simulink model "car_system_SIL_PIL"  (R2019b)
settings: Solver=ode23tb  StartTime=0.0  StopTime=30  RelTol=1e-3
InitFcn:
  | CommonVariables
  | Klqr5Velocities
undefined symbols (not defined in the file): A_1, A_2, A_3, A_4, A_5, B1_1, B1_2, B1_3, B1_4, B1_5, BattChrgMax, BattDischrgMax, BrkPrsMax, ChrgLmt_bpt, Disabled, DischrgLmt_bpt, disk_abore, DLCXref, DLCYref, efficiency_table, F0z, h, Klqr1, Klqr2, Klqr3, Klqr4, Klqr5, MotSpd, MotTrq, mu_kinetic, Ndiff, num_pads, RegenBrkCutOff, RegenBrkSpd_bpt, Right, Rm, SOC_bpt, T_eff_bp, VEH, w_eff_bp
libraries: simulink x10, vehdynlibtire x8, vehdynlibsuspension x7, vehdynlibscenariocommon x5, autolibutils x4, sim3dlib x4, autolibmappedmotor x4, autolibshared x2, sharedtransform x2, vehdynlibviscommon x2, vehdynlibdriver x1, vehdynlibsteering x1
(part 4 of 7)

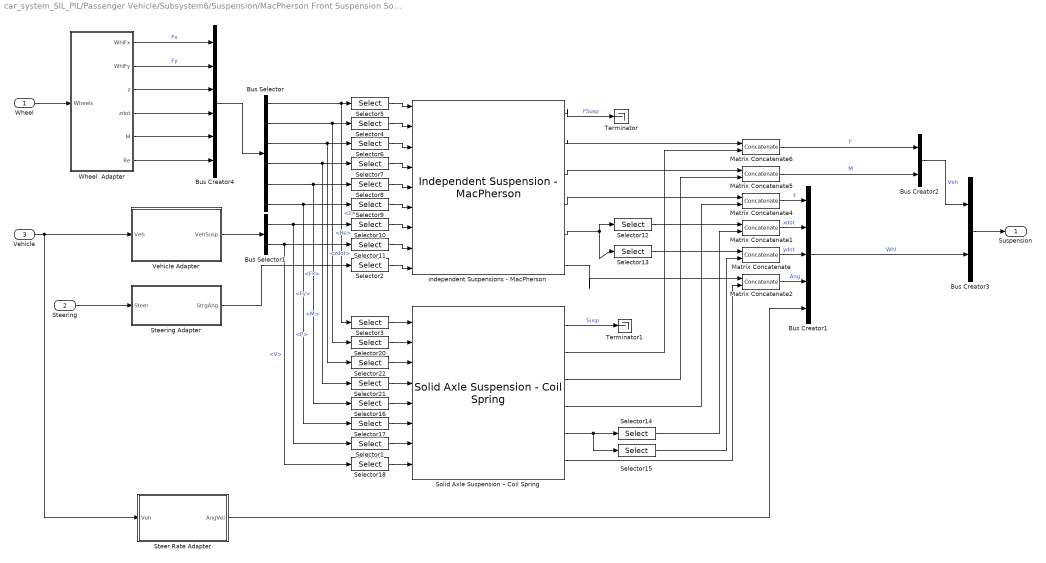
== system car_system_SIL_PIL/Passenger Vehicle/Subsystem6/Suspension/MacPherson Front Suspension Solid Axle Rear Suspension ==
  Wheel : Inport
  Steering : Inport  Port=2
  Vehicle : Inport  Port=3
  Bus Creator1 : BusCreator  Inputs=5
  Bus Creator2 : BusCreator  Inputs=2
  Bus Creator3 : BusCreator  Inputs=2
  Bus Creator4 : BusCreator  Inputs=6
  Bus Selector : BusSelector  OutputSignals=z,Re,zdot,Fx,Fy,M
  Bus Selector1 : BusSelector  OutputSignals=P,V
  Matrix Concatenate{,1..2,4..6} (6 alike) : Concatenate  Mode=Multidimensional array  ConcatenateDimension=2
  Selector1 : Selector  NumberOfDimensions=2  IndexOptions=Select all,Index vector (dialog)  Indices=[1 2],[3 4]  OutputSizes=1,1
  Selector10 : Selector  NumberOfDimensions=2  IndexOptions=Select all,Index vector (dialog)  Indices=[1 2],[1 2]  OutputSizes=1,1
  Selector11 : Selector  NumberOfDimensions=2  IndexOptions=Select all,Index vector (dialog)  Indices=[1 2],[1 2]  OutputSizes=1,1
  Selector12 : Selector  NumberOfDimensions=2  InputPortWidth=3  IndexOptions=Index vector (dialog),Select all  Indices=1,1  OutputSizes=1,1
  Selector13 : Selector  NumberOfDimensions=2  InputPortWidth=3  IndexOptions=Index vector (dialog),Select all  Indices=2,1  OutputSizes=1,1
  Selector14 : Selector  NumberOfDimensions=2  InputPortWidth=3  IndexOptions=Index vector (dialog),Select all  Indices=1,1  OutputSizes=1,1
  Selector15 : Selector  NumberOfDimensions=2  InputPortWidth=3  IndexOptions=Index vector (dialog),Select all  Indices=2,1  OutputSizes=1,1
  Selector{3,16,20..22} (5 alike) : Selector  IndexOptions=Index vector (dialog)  Indices=[3 4]  OutputSizes=1
  Selector17 : Selector  NumberOfDimensions=2  IndexOptions=Select all,Index vector (dialog)  Indices=[1 2],[3 4]  OutputSizes=1,1
  Selector18 : Selector  NumberOfDimensions=2  IndexOptions=Select all,Index vector (dialog)  Indices=[1 2],[3 4]  OutputSizes=1,1
  Selector{2,4..8} (6 alike) : Selector  IndexOptions=Index vector (dialog)  Indices=[1 2]  OutputSizes=1
  Selector9 : Selector  NumberOfDimensions=2  IndexOptions=Select all,Index vector (dialog)  Indices=[1 2],[1 2]  OutputSizes=1,1
  Solid Axle Suspension – Coil Spring : vehdynlibsuspension/Solid Axle Suspension - Coil Spring  NumAxl=1  NumTracksByAxl=2  StrgEnByAxl=0  TrackNumVec="[1  2]"  AxleNumVec="[1  1]"  SuspTypesByAxle=[1]  SuspImage=suspsacoil.png  AxlIxx=AxlIxx  AxlM=AxlM  TrackCoords=[0 0;VEH.TrackWidth*[-1 1]/2;0 0]  SuspCoords=[0 0;VEH.TrackWidth*[-1 1]/2;0 0]  KzWhlAxl=KzWhlAxl  F0zWhlAxl=F0zWhlAxl  CzWhlAxl=CzWhlAxl  IdealSuspEn=on  IdealSuspAxles=[1]  Kz=Kz  F0z=F0z(2)  Cz=Cz  Hmax=Hmax  Toe=0.  RollStrgSlp=0.  ToeStrgSlp=0  Caster=0.  CasterHslp=0.  CasterStrgSlp=0.01  Camber=0.  CamberHslp=0.  CamberStrgSlp=0.01  StrgHgtSlp=0.1432  MappedSuspEn=off  MappedSuspAxles="[1  2]"  f_susp_axl_bp=[1 2]  f_susp_dz_bp=[-0.15 -0.14 -0.13 -0.12 -0.11 -0.10 -0.09 -0.08 -0.07 -0.06 -0.05 -0.04 -0.03 -0.02 -0.01 0.00 0.01 0.02 0.03 0.04 0.05 0.06 0.07 0.08 0.09 0.10 0.11 0.12 0.13 0.14 0.15]  f_susp_dzdot_bp=[-0.15 -0.14 -0.13 -0.12 -0.11 -0.10 -0.09 -0.08 -0.07 -0.06 -0.05 -0.04 -0.03 -0.02 -0.01 0.00 0.01 0.02 0.03 0.04 0.05 0.06 0.07 0.08 0.09 0.10 0.11 0.12 0.13 0.14 0.15]  f_susp_fmz=zeros(31,31,61,2,4)  f_susp_geom=zeros(31,61,2,3)  f_susp_strgdelta_bp=[-30,-29,-28,-27,-26,-25,-24,-23,-22,-21,-20,-19,-18,-17,-16,-15,-14,-13,-12,-11,-10,-9,-8,-7,-6,-5,-4,-3,-2,-1,0,1,2,3,4,5,6,7,8,9,10,11,12,13,14,15,16,17,18,19,20,21,22,23,24,25,26,27,28,29,30]
      settings: SourceProductName=Vehicle Dynamics Blockset  SourceProductBaseCode=VE
  Steer Rate Adapter : Subsystem
  Steering Adapter : Subsystem
  Terminator : Terminator
  Terminator1 : Terminator
  Vehicle Adapter : Subsystem
  Wheel  Adapter : Subsystem
  independent Suspensions - MacPherson : vehdynlibsuspension/Independent Suspension - MacPherson  ActiveDampEn=off  NumAxl=1  NumTracksByAxl=2  StrgEnByAxl=1  AntiSwayEnByAxl=1  TrackNumVec="[1  2]"  AxleNumVec="[1  1]"  SuspTypesByAxle=[1]  SuspImage=suspmacp.png  IdealSuspEn=on  IdealSuspAxles=[1]  Kz=Kz  F0z=F0z(1)  Cz=Cz  Hmax=Hmax  f_act_susp_cz=[10000 10000;10000 10000]  f_act_susp_duty_bpt=[0 1]  f_act_susp_zdot_bpt=[-1 1]  Toe=0.  RollStrgSlp=0.  ToeStrgSlp=0.  Caster=0.  CasterHslp=0.  CasterStrgSlp=0.  Camber=0.  CamberHslp=0.  CamberStrgSlp=0.  StrgHgtSlp=0.1432  MappedSuspEn=off  MappedSuspAxles="[1  2]"  f_susp_axl_bp=[1 2]  f_susp_dz_bp=[-0.15 -0.14 -0.13 -0.12 -0.11 -0.10 -0.09 -0.08 -0.07 -0.06 -0.05 -0.04 -0.03 -0.02 -0.01 0.00 0.01 0.02 0.03 0.04 0.05 0.06 0.07 0.08 0.09 0.10 0.11 0.12 0.13 0.14 0.15]  f_susp_dzdot_bp=[-0.15 -0.14 -0.13 -0.12 -0.11 -0.10 -0.09 -0.08 -0.07 -0.06 -0.05 -0.04 -0.03 -0.02 -0.01 0.00 0.01 0.02 0.03 0.04 0.05 0.06 0.07 0.08 0.09 0.10 0.11 0.12 0.13 0.14 0.15]  f_susp_fmz=zeros(31,31,61,2,4)  f_susp_geom=zeros(31,61,2,3)  f_susp_strgdelta_bp=[-30,-29,-28,-27,-26,-25,-24,-23,-22,-21,-20,-19,-18,-17,-16,-15,-14,-13,-12,-11,-10,-9,-8,-7,-6,-5,-4,-3,-2,-1,0,1,2,3,4,5,6,7,8,9,10,11,12,13,14,15,16,17,18,19,20,21,22,23,24,25,26,27,28,29,30]  AntiSwayR=0.2  AntiSwayNtrlAng=0.5236  AntiSwayTrsK=8e+02
      link override Anti-Sway Force: LabelModeActiveChoice=NoOp
      settings: SourceProductName=Vehicle Dynamics Blockset  SourceProductBaseCode=VE
  Suspension : Outport  VectorParamsAs1DForOutWhenUnconnected=off
  wires:
  Bus Creator3/1 -> Suspension/1
  Bus Creator1/1 -> Bus Creator3/2  "Whl"
  Bus Selector1/2 -> Selector11/1, Selector18/1  "<V>"
  Bus Selector/6 -> Selector9/1, Selector17/1  "<M>"
  Bus Selector/5 -> Selector8/1, Selector16/1  "<Fy>"
  Bus Selector/1 -> Selector3/1, Selector5/1  "<z>"
  Steering/1 -> Steering Adapter/1(Steer)
  Bus Selector1/1 -> Selector10/1, Selector1/1  "<P>"
  Matrix Concatenate/1 -> Bus Creator1/3  "ydot"
  independent Suspensions - MacPherson/5 -> Selector12/1, Selector13/1
  independent Suspensions - MacPherson/6 -> Matrix Concatenate2/1
  Selector12/1 -> Matrix Concatenate1/1
  independent Suspensions - MacPherson/4 -> Matrix Concatenate4/1
  independent Suspensions - MacPherson/1 -> Terminator/1  "FSusp"
  Bus Selector/4 -> Selector7/1, Selector21/1  "<Fx>"
  Vehicle Adapter/1(VehSusp) -> Bus Selector1/1
  independent Suspensions - MacPherson/2 -> Matrix Concatenate6/1
  independent Suspensions - MacPherson/3 -> Matrix Concatenate5/1
  Bus Creator2/1 -> Bus Creator3/1  "Veh"
  Steering Adapter/1(StrgAng) -> Selector2/1
  Bus Creator4/1 -> Bus Selector/1
  Wheel  Adapter/2(WhlFy) -> Bus Creator4/2  "Fy"
  Wheel  Adapter/1(WhlFx) -> Bus Creator4/1  "Fx"
  Wheel/1 -> Wheel  Adapter/1(Wheels)
  Wheel  Adapter/3(z) -> Bus Creator4/3
  Wheel  Adapter/4(zdot) -> Bus Creator4/4
  Wheel  Adapter/5(M) -> Bus Creator4/5
  Bus Selector/2 -> Selector20/1, Selector4/1  "<Re>"
  Selector2/1 -> independent Suspensions - MacPherson/9
  Selector3/1 -> Solid Axle Suspension – Coil Spring/1
  Selector4/1 -> independent Suspensions - MacPherson/2
  Selector5/1 -> independent Suspensions - MacPherson/1
  Selector6/1 -> independent Suspensions - MacPherson/3
  Selector7/1 -> independent Suspensions - MacPherson/4
  Selector8/1 -> independent Suspensions - MacPherson/5
  Selector9/1 -> independent Suspensions - MacPherson/6
  Selector10/1 -> independent Suspensions - MacPherson/7
  Selector11/1 -> independent Suspensions - MacPherson/8
  Selector13/1 -> Matrix Concatenate/1
  Selector15/1 -> Matrix Concatenate/2
  Matrix Concatenate1/1 -> Bus Creator1/2  "xdot"
  Selector14/1 -> Matrix Concatenate1/2
  Matrix Concatenate2/1 -> Bus Creator1/4  "Ang"
  Solid Axle Suspension – Coil Spring/6 -> Matrix Concatenate2/2
  Matrix Concatenate4/1 -> Bus Creator1/1  "F"
  Solid Axle Suspension – Coil Spring/4 -> Matrix Concatenate4/2
  Matrix Concatenate5/1 -> Bus Creator2/2  "M"
  Matrix Concatenate6/1 -> Bus Creator2/1  "F"
  Solid Axle Suspension – Coil Spring/2 -> Matrix Concatenate6/2
  Selector16/1 -> Solid Axle Suspension – Coil Spring/5
  Selector17/1 -> Solid Axle Suspension – Coil Spring/6
  Selector1/1 -> Solid Axle Suspension – Coil Spring/7
  Selector18/1 -> Solid Axle Suspension – Coil Spring/8
  Selector20/1 -> Solid Axle Suspension – Coil Spring/2
  Wheel  Adapter/6(Re) -> Bus Creator4/6
  Selector21/1 -> Solid Axle Suspension – Coil Spring/4
  Solid Axle Suspension – Coil Spring/3 -> Matrix Concatenate5/2
  Vehicle/1 -> Steer Rate Adapter/1(Veh), Vehicle Adapter/1(Veh)
  Selector22/1 -> Solid Axle Suspension – Coil Spring/3
  Bus Selector/3 -> Selector22/1, Selector6/1  "<zdot>"
  Solid Axle Suspension – Coil Spring/1 -> Terminator1/1  "Susp"
  Solid Axle Suspension – Coil Spring/5 -> Selector15/1, Selector14/1
  Steer Rate Adapter/1(AngVel) -> Bus Creator1/5

== system car_system_SIL_PIL/Passenger Vehicle/Subsystem6/Suspension/MacPherson Suspension ==
  Wheel : Inport
  Steering : Inport  Port=2
  Vehicle : Inport  Port=3
  Bus Creator1 : BusCreator  Inputs=5
  Bus Creator2 : BusCreator  Inputs=2
  Bus Creator3 : BusCreator  Inputs=2
  Bus Creator4 : BusCreator  Inputs=6
  Bus Selector : BusSelector  OutputSignals=z,Re,zdot,Fx,Fy,M
  Bus Selector1 : BusSelector  OutputSignals=P,V
  Selector1 : Selector  NumberOfDimensions=2  IndexOptions=Index vector (dialog),Select all  Indices=1,1  OutputSizes=1,1
  Selector2 : Selector  NumberOfDimensions=2  IndexOptions=Index vector (dialog),Select all  Indices=2,1  OutputSizes=1,1
  Steer Rate Adapter : Subsystem
  Steering Adapter : Subsystem
  Terminator : Terminator
  Vehicle Adapter : Subsystem
  Wheel  Adapter : Subsystem
  independent Suspensions - MacPherson : vehdynlibsuspension/Independent Suspension - MacPherson  ActiveDampEn=off  NumAxl=2  NumTracksByAxl=[2 2]  StrgEnByAxl=[1 0]  AntiSwayEnByAxl=[1 0]  TrackNumVec="[1  2  1  2]"  AxleNumVec="[1  1  2  2]"  SuspTypesByAxle="[1  1]"  SuspImage=suspmacp.png  IdealSuspEn=on  IdealSuspAxles="[1  2]"  Kz=Kz  F0z=F0z  Cz=Cz  Hmax=Hmax  f_act_susp_cz=[10000 10000;10000 10000]  f_act_susp_duty_bpt=[0 1]  f_act_susp_zdot_bpt=[-1 1]  Toe=0.  RollStrgSlp=0.  ToeStrgSlp=0.  Caster=0.  CasterHslp=0.  CasterStrgSlp=0.  Camber=0.  CamberHslp=0.  CamberStrgSlp=0.  StrgHgtSlp=0.1432  MappedSuspEn=off  MappedSuspAxles="[1  2]"  f_susp_axl_bp=[1 2]  f_susp_dz_bp=[-0.15 -0.14 -0.13 -0.12 -0.11 -0.10 -0.09 -0.08 -0.07 -0.06 -0.05 -0.04 -0.03 -0.02 -0.01 0.00 0.01 0.02 0.03 0.04 0.05 0.06 0.07 0.08 0.09 0.10 0.11 0.12 0.13 0.14 0.15]  f_susp_dzdot_bp=[-0.15 -0.14 -0.13 -0.12 -0.11 -0.10 -0.09 -0.08 -0.07 -0.06 -0.05 -0.04 -0.03 -0.02 -0.01 0.00 0.01 0.02 0.03 0.04 0.05 0.06 0.07 0.08 0.09 0.10 0.11 0.12 0.13 0.14 0.15]  f_susp_fmz=zeros(31,31,61,2,4)  f_susp_geom=zeros(31,61,2,3)  f_susp_strgdelta_bp=[-30,-29,-28,-27,-26,-25,-24,-23,-22,-21,-20,-19,-18,-17,-16,-15,-14,-13,-12,-11,-10,-9,-8,-7,-6,-5,-4,-3,-2,-1,0,1,2,3,4,5,6,7,8,9,10,11,12,13,14,15,16,17,18,19,20,21,22,23,24,25,26,27,28,29,30]  AntiSwayR=0.2  AntiSwayNtrlAng=0.5236  AntiSwayTrsK=8e+02
      settings: SourceProductName=Vehicle Dynamics Blockset  SourceProductBaseCode=VE
  Suspension : Outport  VectorParamsAs1DForOutWhenUnconnected=off
  wires:
  Bus Creator3/1 -> Suspension/1
  Bus Creator1/1 -> Bus Creator3/2  "Whl"
  Bus Selector1/2 -> independent Suspensions - MacPherson/8  "<V>"
  Bus Selector/6 -> independent Suspensions - MacPherson/6  "<M>"
  Bus Selector/5 -> independent Suspensions - MacPherson/5  "<Fy>"
  Steering/1 -> Steering Adapter/1(Steer)
  Bus Selector/3 -> independent Suspensions - MacPherson/3  "<zdot>"
  Bus Selector/4 -> independent Suspensions - MacPherson/4  "<Fx>"
  Vehicle/1 -> Steer Rate Adapter/1(Veh), Vehicle Adapter/1(Veh)
  Vehicle Adapter/1(VehSusp) -> Bus Selector1/1
  independent Suspensions - MacPherson/3 -> Bus Creator2/2  "M"
  Wheel  Adapter/2(WhlFy) -> Bus Creator4/2  "Fy"
  Wheel  Adapter/1(WhlFx) -> Bus Creator4/1  "Fx"
  Wheel/1 -> Wheel  Adapter/1(Wheels)
  Wheel  Adapter/3(z) -> Bus Creator4/3
  Wheel  Adapter/4(zdot) -> Bus Creator4/4
  Wheel  Adapter/5(M) -> Bus Creator4/5  "M"
  Wheel  Adapter/6(Re) -> Bus Creator4/6
  Bus Selector/2 -> independent Suspensions - MacPherson/2  "<Re>"
  Selector1/1 -> Bus Creator1/2  "xdot"
  Selector2/1 -> Bus Creator1/3  "ydot"
  Bus Selector1/1 -> independent Suspensions - MacPherson/7  "<P>"
  Bus Selector/1 -> independent Suspensions - MacPherson/1  "<z>"
  independent Suspensions - MacPherson/4 -> Bus Creator1/1  "F"
  independent Suspensions - MacPherson/6 -> Bus Creator1/4  "Ang"
  independent Suspensions - MacPherson/5 -> Selector2/1, Selector1/1  "V"
  independent Suspensions - MacPherson/2 -> Bus Creator2/1  "F"
  Bus Creator2/1 -> Bus Creator3/1  "Veh"
  Bus Creator4/1 -> Bus Selector/1
  Steer Rate Adapter/1(AngVel) -> Bus Creator1/5  "AngVel"
  Steering Adapter/1(StrgAng) -> independent Suspensions - MacPherson/9
  independent Suspensions - MacPherson/1 -> Terminator/1  "Susp"

== system car_system_SIL_PIL/Passenger Vehicle/Subsystem6/Suspension/Mapped Suspension ==
  Wheel : Inport
  Steering : Inport  Port=2
  Vehicle : Inport  Port=3
  Bus Creator1 : BusCreator  Inputs=5
  Bus Creator2 : BusCreator  Inputs=2
  Bus Creator3 : BusCreator  Inputs=2
  Bus Creator4 : BusCreator  Inputs=6
  Bus Selector : BusSelector  OutputSignals=z,Re,zdot,Fx,Fy,M
  Bus Selector1 : BusSelector  OutputSignals=P,V
  Independent Suspension - Mapped : vehdynlibsuspension/Independent Suspension - Mapped  NumAxl=2  NumTracksByAxl=[2 2]  StrgEnByAxl=[1 0]  AntiSwayEnByAxl=[1 0]  TrackNumVec="[1  2  1  2]"  AxleNumVec="[1  1  2  2]"  SuspTypesByAxle="[2  2]"  SuspImage=suspindmap.png  IdealSuspEn=off  IdealSuspAxles="[1  2]"  Kz=64370  F0z=9810  Cz=10000  Hmax=0.5  Toe=2  RollStrgSlp=-13  ToeStrgSlp=0.01  Caster=4  CasterHslp=-13  CasterStrgSlp=0.01  Camber=4  CamberHslp=-13  CamberStrgSlp=0.01  StrgHgtSlp=0.0025  MappedSuspEn=on  MappedSuspAxles="[1  2]"  f_susp_axl_bp=[1 2]  f_susp_dz_bp=f_susp_dz_bp  f_susp_dzdot_bp=f_susp_dzdot_bp  f_susp_fmz=f_susp_fmz  f_susp_geom=f_susp_geom  f_susp_strgdelta_bp=f_susp_strgdelta_bp  NDFLookupOutType=1:4  NDGLookupOutType=1:3  AntiSwayR=0.2  AntiSwayNtrlAng=0.5236  AntiSwayTrsK=8e2
      link override For each track and axle combination calculate suspension forces and moments/Suspension/Suspension Angle Calculations: OverrideUsingVariant=MappedSteeringEnabled
      link override For each track and axle combination calculate suspension forces and moments/Suspension/Z axis suspension characteristic: OverrideUsingVariant=MappedSuspension
      settings: SourceProductName=Vehicle Dynamics Blockset  SourceProductBaseCode=VE
  Reshape1 : Reshape  OutputDimensionality=Row vector (2-D)
  Selector : Selector  IndexOptions=Index vector (dialog)  Indices=[1 2]  OutputSizes=1
  Selector1 : Selector  NumberOfDimensions=2  IndexOptions=Index vector (dialog),Select all  Indices=1,1  OutputSizes=1,1
  Selector2 : Selector  NumberOfDimensions=2  IndexOptions=Index vector (dialog),Select all  Indices=2,1  OutputSizes=1,1
  Steer Rate Adapter : Subsystem
  Terminator : Terminator
  Vehicle Adapter : Subsystem
  Wheel  Adapter : Subsystem
  Suspension : Outport  VectorParamsAs1DForOutWhenUnconnected=off
  wires:
  Independent Suspension - Mapped/1 -> Terminator/1  "Susp"
  Reshape1/1 -> Independent Suspension - Mapped/9
  Bus Selector/5 -> Independent Suspension - Mapped/5  "<Fy>"
  Bus Selector/2 -> Independent Suspension - Mapped/2  "<Re>"
  Bus Selector1/2 -> Independent Suspension - Mapped/8  "<V>"
  Bus Selector/4 -> Independent Suspension - Mapped/4  "<Fx>"
  Wheel  Adapter/5(M) -> Bus Creator4/5
  Bus Selector/6 -> Independent Suspension - Mapped/6  "<M>"
  Wheel  Adapter/4(zdot) -> Bus Creator4/4
  Wheel  Adapter/6(Re) -> Bus Creator4/6
  Selector/1 -> Reshape1/1
  Bus Creator4/1 -> Bus Selector/1
  Wheel  Adapter/3(z) -> Bus Creator4/3
  Wheel  Adapter/2(WhlFy) -> Bus Creator4/2  "Fy"
  Wheel/1 -> Wheel  Adapter/1(Wheels)
  Vehicle Adapter/1(VehSusp) -> Bus Selector1/1
  Bus Selector/3 -> Independent Suspension - Mapped/3  "<zdot>"
  Bus Selector/1 -> Independent Suspension - Mapped/1  "<z>"
  Wheel  Adapter/1(WhlFx) -> Bus Creator4/1  "Fx"
  Bus Selector1/1 -> Independent Suspension - Mapped/7  "<P>"
  Steering/1 -> Selector/1
  Vehicle/1 -> Steer Rate Adapter/1(Veh), Vehicle Adapter/1(Veh)
  Independent Suspension - Mapped/6 -> Bus Creator1/4  "Ang"
  Selector2/1 -> Bus Creator1/3  "ydot"
  Independent Suspension - Mapped/2 -> Bus Creator2/1  "F"
  Independent Suspension - Mapped/3 -> Bus Creator2/2  "M"
  Bus Creator2/1 -> Bus Creator3/1  "Veh"
  Bus Creator1/1 -> Bus Creator3/2  "Whl"
  Independent Suspension - Mapped/4 -> Bus Creator1/1  "F"
  Selector1/1 -> Bus Creator1/2  "xdot"
  Independent Suspension - Mapped/5 -> Selector2/1, Selector1/1  "V"
  Bus Creator3/1 -> Suspension/1
  Steer Rate Adapter/1(AngVel) -> Bus Creator1/5

== system car_system_SIL_PIL/Passenger Vehicle/Subsystem6/Vehicle/Variant Subsystem ==
  note: 1) Add Subsystem or Model blocks as valid variant choices.
      | 2) You cannot connect blocks at this level. At simulation, connectivity is automatically
      | determined, based on the active variant and port name matching.
  Suspension : Inport
  Wind : Inport  Port=2
  3DOF : Subsystem  VariantControl=0
  6DOF : Subsystem  VariantControl=1
  VehFdbk : Outport  VectorParamsAs1DForOutWhenUnconnected=off

== system car_system_SIL_PIL/Passenger Vehicle/Subsystem6/Wheels and Tires/VDBS ==
  WheelAng : Inport
  CamberAng : Inport  Port=2  Unit=rad
  AxleTrq : Inport  Port=3
  BrkPrs : Inport  Port=4
  Fz : Inport  Port=5  Unit=N
  r : Inport  Port=6
  VehVel : Inport  Port=7
  Ground Level : Inport  Port=8
  Friction : Inport  Port=9  Unit=1  PortDimensions=4
  Pressure : vehdynlibtirecommon/Constant  const=220000  numWheels=4
      settings: SourceProductName=Vehicle Dynamics Blockset  SourceProductBaseCode=VE
  Terminator : Terminator
  Tire2Veh : Subsystem
  Tires : Subsystem  VariantControlMode=Label  Variant=on  VariantControl=Variant1  LabelModeActiveChoice=0
  Veh2Tire : Subsystem
  scale factors with friction : Subsystem  mask{numWheels=4}
      mask prompts: numWheels "Number of wheels"
  Wheels : Outport  VectorParamsAs1DForOutWhenUnconnected=off
  FrntAxlF : Outport  Port=2  Unit=N  VectorParamsAs1DForOutWhenUnconnected=off
  RearAxlF : Outport  Port=3  Unit=N  VectorParamsAs1DForOutWhenUnconnected=off
  omega : Outport  Port=4  VectorParamsAs1DForOutWhenUnconnected=off
  SteerTrq : Outport  Port=5  Unit=N*m  VectorParamsAs1DForOutWhenUnconnected=off
  SuspWhlPz : Outport  Port=6  VectorParamsAs1DForOutWhenUnconnected=off
  SuspWhlVz : Outport  Port=7  VectorParamsAs1DForOutWhenUnconnected=off
  wires:
  Ground Level/1 -> Tires/9("Gnd ")
  Pressure/1 -> Tires/7("Press ")
  scale factors with friction/1(lambdas) -> Tires/8("lambda ")
  Fz/1 -> Tires/10("FzSusp "), Tire2Veh/2(Fz)
  AxleTrq/1 -> Veh2Tire/2(Axle)
  BrkPrs/1 -> Veh2Tire/3(Brake)
  VehVel/1 -> Veh2Tire/4(VehVel)
  Veh2Tire/1(T) -> Tires/1("DriveTorque ")
  Veh2Tire/2(P) -> Tires/2("Brake Pressure ")
  Veh2Tire/4(xdotAxle) -> Tires/4("Vx ")
  Veh2Tire/5(ydotAxle) -> Tires/5("Vy ")
  Veh2Tire/3(psidot) -> Tires/3("r ")
  Tires/1(" Wheels") -> Tire2Veh/1(Wheel)
  WheelAng/1 -> Veh2Tire/5(WheelSteer), Tire2Veh/4(WheelSteer)
  Tire2Veh/2(Out3) -> omega/1
  Tire2Veh/3(Out4) -> FrntAxlF/1
  Tire2Veh/4(Out5) -> RearAxlF/1
  Tire2Veh/5(<Mz>) -> SteerTrq/1
  Friction/1 -> scale factors with friction/2(lamda_mu_y), scale factors with friction/1(lamda_mu_x)
  r/1 -> Veh2Tire/1(r)
  Veh2Tire/6(zdotAxle) -> Terminator/1
  Tire2Veh/6(SuspWhlPz) -> SuspWhlPz/1
  Tire2Veh/7(SuspWhlVz) -> SuspWhlVz/1
  CamberAng/1 -> Tires/6("Camber "), Tire2Veh/3(WheelCamber), Veh2Tire/6(WheelCamber)
  Tire2Veh/1(Wheels) -> Wheels/1  "TireFrame"

== system car_system_SIL_PIL/Reference Generator/3D Engine/3D Engine/Part Rotation Concatenation ==
  Body Roll : Inport
  Body Ptich : Inport  Port=2
  Body Yaw : Inport  Port=3
  WheelFrontLeft Pitch : Inport  Port=4
  WheelFrontRight Pitch : Inport  Port=5
  WheelRearLeft Pitch : Inport  Port=6
  WheelRearRight Ptich : Inport  Port=7
  WheelFrontLeft Roll : Inport  Port=8
  WheelFrontRight Roll : Inport  Port=9
  WheelRearLeft Roll : Inport  Port=10
  WheelRearRight Roll : Inport  Port=11
  WheelFrontLeft Yaw : Inport  Port=12
  WheelFrontRight Yaw : Inport  Port=13
  WheelRearLeft Yaw : Inport  Port=14
  WheelRearRight Yaw : Inport  Port=15
  AllParts : Concatenate  NumInputs=5  Mode=Multidimensional array
  Body : Concatenate  NumInputs=3  Mode=Multidimensional array  ConcatenateDimension=2
  WheelFrontLeft : Concatenate  NumInputs=3  Mode=Multidimensional array  ConcatenateDimension=2
  WheelFrontRight : Concatenate  NumInputs=3  Mode=Multidimensional array  ConcatenateDimension=2
  WheelRearLeft : Concatenate  NumInputs=3  Mode=Multidimensional array  ConcatenateDimension=2
  WheelRearRight : Concatenate  NumInputs=3  Mode=Multidimensional array  ConcatenateDimension=2
  ConcatOut : Outport  VectorParamsAs1DForOutWhenUnconnected=off
  wires:
  Body Ptich/1 -> Body/1
  Body Yaw/1 -> Body/3
  WheelFrontLeft Pitch/1 -> WheelFrontLeft/1
  WheelFrontLeft Yaw/1 -> WheelFrontLeft/3
  WheelFrontLeft Roll/1 -> WheelFrontLeft/2
  Body Roll/1 -> Body/2
  WheelFrontLeft/1 -> AllParts/2
  WheelRearRight Ptich/1 -> WheelRearRight/1
  Body/1 -> AllParts/1
  WheelRearLeft/1 -> AllParts/4
  WheelFrontRight/1 -> AllParts/3
  WheelRearRight Yaw/1 -> WheelRearRight/3
  WheelFrontRight Roll/1 -> WheelFrontRight/2
  WheelFrontRight Pitch/1 -> WheelFrontRight/1
  WheelRearRight Roll/1 -> WheelRearRight/2
  WheelRearLeft Yaw/1 -> WheelRearLeft/3
  AllParts/1 -> ConcatOut/1
  WheelRearLeft Roll/1 -> WheelRearLeft/2
  WheelRearRight/1 -> AllParts/5
  WheelRearLeft Pitch/1 -> WheelRearLeft/1
  WheelFrontRight Yaw/1 -> WheelFrontRight/3

== system car_system_SIL_PIL/Reference Generator/3D Engine/3D Engine/Part Translation Concatenation ==
  BodyX : Inport
  BodyY : Inport  Port=2
  BodyZ : Inport  Port=3
  WheelFrontLeftX : Inport  Port=4
  WheelFrontRightX : Inport  Port=5
  WheelRearLeftX : Inport  Port=6
  WheelRearRightX : Inport  Port=7
  WheelFrontLeftY : Inport  Port=8
  WheelFrontRightY : Inport  Port=9
  WheelRearLeftY : Inport  Port=10
  WheelRearRightY : Inport  Port=11
  WheelFrontLeftZ : Inport  Port=12
  WheelFrontRightZ : Inport  Port=13
  WheelRearLeftZ : Inport  Port=14
  WheelRearRightZ : Inport  Port=15
  AllParts : Concatenate  NumInputs=5  Mode=Multidimensional array
  Body : Concatenate  NumInputs=3  Mode=Multidimensional array  ConcatenateDimension=2
  WheelFrontLeft : Concatenate  NumInputs=3  Mode=Multidimensional array  ConcatenateDimension=2
  WheelFrontRight : Concatenate  NumInputs=3  Mode=Multidimensional array  ConcatenateDimension=2
  WheelRearLeft : Concatenate  NumInputs=3  Mode=Multidimensional array  ConcatenateDimension=2
  WheelRearRight : Concatenate  NumInputs=3  Mode=Multidimensional array  ConcatenateDimension=2
  ConcatOut : Outport  VectorParamsAs1DForOutWhenUnconnected=off
  wires:
  BodyX/1 -> Body/1
  BodyZ/1 -> Body/3
  WheelFrontLeftX/1 -> WheelFrontLeft/1
  WheelFrontLeftZ/1 -> WheelFrontLeft/3
  WheelFrontLeftY/1 -> WheelFrontLeft/2
  BodyY/1 -> Body/2
  WheelFrontLeft/1 -> AllParts/2
  WheelRearRightX/1 -> WheelRearRight/1
  Body/1 -> AllParts/1
  WheelRearLeft/1 -> AllParts/4
  WheelFrontRight/1 -> AllParts/3
  WheelRearRightZ/1 -> WheelRearRight/3
  WheelFrontRightY/1 -> WheelFrontRight/2
  WheelFrontRightX/1 -> WheelFrontRight/1
  WheelRearRightY/1 -> WheelRearRight/2
  WheelRearLeftZ/1 -> WheelRearLeft/3
  AllParts/1 -> ConcatOut/1
  WheelRearLeftY/1 -> WheelRearLeft/2
  WheelRearRight/1 -> AllParts/5
  WheelRearLeftX/1 -> WheelRearLeft/1
  WheelFrontRightZ/1 -> WheelFrontRight/3

== system car_system_SIL_PIL/Reference Generator/3D Engine/3D Engine/Scale ==
  Constant{1..12,17,32..33} (15 alike) : Constant  OutDataTypeStr=single
  PartConcatenation : Subsystem
  ScaleOut : Outport  VectorParamsAs1DForOutWhenUnconnected=off
  wires:
  Constant10/1 -> PartConcatenation/15(WheelRearRightZ)
  Constant9/1 -> PartConcatenation/14(WheelRearRightY)
  Constant11/1 -> PartConcatenation/13(WheelRearRightX)
  Constant7/1 -> PartConcatenation/12(WheelRearLeftZ)
  Constant6/1 -> PartConcatenation/11(WheelRearLeftY)
  Constant8/1 -> PartConcatenation/10(WheelRearLeftX)
  Constant4/1 -> PartConcatenation/9(WheelFrontRightZ)
  Constant3/1 -> PartConcatenation/8(WheelFrontRightY)
  Constant5/1 -> PartConcatenation/7(WheelFrontRightX)
  Constant2/1 -> PartConcatenation/6(WheelFrontLeftZ)
  Constant1/1 -> PartConcatenation/5(WheelFrontLeftY)
  Constant33/1 -> PartConcatenation/4(WheelFrontLeftX)
  Constant32/1 -> PartConcatenation/3(BodyZ)
  Constant17/1 -> PartConcatenation/2(BodyY)
  Constant12/1 -> PartConcatenation/1(BodyX)
  PartConcatenation/1(ConcatOut) -> ScaleOut/1

== system car_system_SIL_PIL/Reference Generator/3D Engine/3D Engine/VehicleActorTransform 2 ==
  Constant : Constant  Value=[0 0 depth; 0 0 0; 0 0 0; 0 0 0; 0 0 0]
  Constant1 : Constant  Value=[0 0 0; 0 0 0; 0 0 0; 0 0 0; 0 0 0]
  Constant2 : Constant  Value=ones(5,3)
  Vehicle Actor Transform Set1 : sim3dlib/Simulation 3D Actor Transform Set  ActorTag=SimulinkVehicle2  ActorType=Passenger vehicle  PassVehMesh=Muscle car  VehColor=Green  NumberOfParts=5  CustNumOfParts=3  Translation=[0 0 depth; 0 0 0; 0 0 0; 0 0 0; 0 0 0]  Rotation=[0 0 0; 0 0 0; 0 0 0; 0 0 0; 0 0 0]  Scale=[1 1 1; 1 1 1; 1 1 1; 1 1 1; 1 1 1]  Ts=-1  aMode=aMode
      settings: SourceProductName=Vehicle Dynamics Blockset  SourceProductBaseCode=VE
  wires:
  Constant/1 -> Vehicle Actor Transform Set1/1
  Constant2/1 -> Vehicle Actor Transform Set1/3
  Constant1/1 -> Vehicle Actor Transform Set1/2

== system car_system_SIL_PIL/Reference Generator/Reference Generator/Constant Radius/Constant Radius ==
  XVeh : Inport
  YVeh : Inport  Port=2
  psiVeh : Inport  Port=3
  Constant : Constant  Value=0
  Constant5 : Constant
  Demux : Demux  Outputs=3
  Demux1 : Demux  Outputs=3
  MATLAB Function : MATLAB Function  TreatAsAtomicUnit=on
  Mux : Mux  Inputs=3
  Mux1 : Mux  Inputs=3
  R : Constant  Value=Value
  Signal Specification{1..4} (4 alike) : SignalSpecification  Unit=m
  Switch : Switch  Criteria=u2 > Threshold
  Terminator1 : Terminator
  Unit Delay : UnitDelay  SampleTime=-1  HasFrameUpgradeWarning=on
  Unit Delay1 : UnitDelay  SampleTime=-1  HasFrameUpgradeWarning=on
  yRef : Outport  VectorParamsAs1DForOutWhenUnconnected=off
  yFdbk : Outport  Port=2  VectorParamsAs1DForOutWhenUnconnected=off
  XRef : Outport  Port=3  VectorParamsAs1DForOutWhenUnconnected=off
  YRef : Outport  Port=4  VectorParamsAs1DForOutWhenUnconnected=off
  wires:
  Signal Specification4/1 -> yFdbk/1
  MATLAB Function/2(yFdbk) -> Signal Specification4/1
  MATLAB Function/3(VehRef) -> Demux1/1
  Signal Specification3/1 -> yRef/1
  MATLAB Function/1(yRef) -> Signal Specification3/1
  Signal Specification2/1 -> XRef/1
  Signal Specification1/1 -> YRef/1
  Demux1/1 -> Signal Specification2/1
  Demux1/2 -> Signal Specification1/1
  Demux1/3 -> Terminator1/1
  psiVeh/1 -> Mux1/3
  R/1 -> MATLAB Function/1(Rref)
  Unit Delay/1 -> Switch/1
  Mux1/1 -> Switch/3
  Unit Delay1/1 -> Switch/2
  Constant/1 -> Mux/3
  Switch/1 -> Unit Delay/1, Demux/1
  Demux/1 -> MATLAB Function/3(Xo)
  Demux/3 -> MATLAB Function/5(psio)
  XVeh/1 -> Mux1/1, Mux/1
  Demux/2 -> MATLAB Function/4(Yo)
  YVeh/1 -> Mux1/2, Mux/2
  Constant5/1 -> Unit Delay1/1
  Mux/1 -> MATLAB Function/2(InertCGDisp)

== system car_system_SIL_PIL/Reference Generator/Reference Generator/Constant Radius/Longitudinal Velocity Reference ==
  Input Units : SignalSpecification  Unit=mph
  Ramp1 : simulink/Sources/Ramp  slope=5  start=t_start  InitialOutput=0
  Saturation1 : Saturate  UpperLimit=xdot_r  LowerLimit=0  ZeroCross=off
  Signal Specification1 : SignalSpecification  Unit=m/s
  Unit Conversion1 : UnitConversion
  xdot : Outport  VectorParamsAs1DForOutWhenUnconnected=off
  wires:
  Unit Conversion1/1 -> Signal Specification1/1
  Signal Specification1/1 -> xdot/1
  Saturation1/1 -> Input Units/1
  Ramp1/1 -> Saturation1/1
  Input Units/1 -> Unit Conversion1/1

== system car_system_SIL_PIL/Visualization/Vehicle XY Plotter/XY View/Vehicle XY Plotter ==
  InertXYZ : Inport
  InertAng : Inport  Port=2
  InertXdotYdotZdot : Inport  Port=3
  delta : Inport  Port=4
  Rate Transition{1..5} (5 alike) : RateTransition  Deterministic=off  OutPortSampleTime=pltDT
  RefXYZ Ground : Ground
  Vehicle XY Plotter : vehdynlibviscommon/Vehicle XY Plotter  bufferSize=bufferSize  w=w  a=a  b=b  figBorder=figBorder
      settings: SourceProductName=Vehicle Dynamics Blockset  SourceProductBaseCode=VE
  wires:
  Rate Transition5/1 -> Vehicle XY Plotter/4
  Rate Transition4/1 -> Vehicle XY Plotter/3
  Rate Transition2/1 -> Vehicle XY Plotter/2
  Rate Transition1/1 -> Vehicle XY Plotter/1
  Rate Transition3/1 -> Vehicle XY Plotter/5
  delta/1 -> Rate Transition5/1  "delta"
  InertXYZ/1 -> Rate Transition1/1  "InertCGDisp"
  InertXdotYdotZdot/1 -> Rate Transition4/1  "InertCGVel"
  InertAng/1 -> Rate Transition2/1  "InertCGDisp"
  RefXYZ Ground/1 -> Rate Transition3/1

== system car_system_SIL_PIL/Visualization/Vehicle XY Plotter/XY View Ref/Vehicle XY Plotter ==
  InertXYZ : Inport
  InertAng : Inport  Port=2
  InertXdotYdotZdot : Inport  Port=3
  delta : Inport  Port=4
  RefXYZ : Inport  Port=5
  Rate Transition{1..5} (5 alike) : RateTransition  Deterministic=off  OutPortSampleTime=pltDT
  Vehicle XY Plotter : vehdynlibviscommon/Vehicle XY Plotter  bufferSize=bufferSize  w=w  a=a  b=b  figBorder=figBorder
      settings: SourceProductName=Vehicle Dynamics Blockset  SourceProductBaseCode=VE
  wires:
  InertAng/1 -> Rate Transition2/1  "InertCGDisp"
  InertXdotYdotZdot/1 -> Rate Transition4/1  "InertCGVel"
  InertXYZ/1 -> Rate Transition1/1  "InertCGDisp"
  delta/1 -> Rate Transition5/1  "delta"
  Rate Transition3/1 -> Vehicle XY Plotter/5
  Rate Transition1/1 -> Vehicle XY Plotter/1
  Rate Transition2/1 -> Vehicle XY Plotter/2
  Rate Transition4/1 -> Vehicle XY Plotter/3
  Rate Transition5/1 -> Vehicle XY Plotter/4
  RefXYZ/1 -> Rate Transition3/1

== system car_system_SIL_PIL/Passenger Vehicle/Subsystem6/Suspension/Double Wishbone Suspension/Steer Rate Adapter ==
  Veh : Inport
  Add : Sum
  Bus Selector3 : BusSelector  OutputSignals=BdyFrm.Cg.AngVel.r
  Constant : Constant  Value=zeros(1,4)
  Matrix Concatenate : Concatenate  NumInputs=3  Mode=Multidimensional array
  Matrix Concatenate1 : Concatenate  NumInputs=3  Mode=Multidimensional array
  Reshape2 : Reshape  OutputDimensionality=Row vector (2-D)
  Reshape3 : Reshape  OutputDimensionality=Row vector (2-D)
  Reshape4 : Reshape  OutputDimensionality=Row vector (2-D)
  Selector3 : Selector  InputPortWidth=1  IndexOptions=Index vector (dialog)  Indices=[1 1 1 1]  OutputSizes=1
  SteerRates : Constant  Value=zeros(1,4)
  AngVel : Outport  VectorParamsAs1DForOutWhenUnconnected=off
  wires:
  Reshape2/1 -> Matrix Concatenate1/1, Matrix Concatenate1/3, Matrix Concatenate1/2
  Constant/1 -> Reshape3/1
  Selector3/1 -> Reshape4/1
  Bus Selector3/1 -> Selector3/1  "<r>"
  Matrix Concatenate/1 -> Add/2
  SteerRates/1 -> Reshape2/1
  Reshape4/1 -> Matrix Concatenate/3
  Reshape3/1 -> Matrix Concatenate/2, Matrix Concatenate/1
  Matrix Concatenate1/1 -> Add/1
  Veh/1 -> Bus Selector3/1
  Add/1 -> AngVel/1  "AngVel"

== system car_system_SIL_PIL/Passenger Vehicle/Subsystem6/Suspension/Double Wishbone Suspension/Steering Adapter ==
  Steer : Inport
  Reshape1 : Reshape  OutputDimensionality=Row vector (2-D)
  Selector : Selector  IndexOptions=Index vector (dialog)  Indices=[1 2]  OutputSizes=1
  StrgAng : Outport  VectorParamsAs1DForOutWhenUnconnected=off
  wires:
  Reshape1/1 -> StrgAng/1
  Steer/1 -> Selector/1
  Selector/1 -> Reshape1/1

== system car_system_SIL_PIL/Passenger Vehicle/Subsystem6/Suspension/Double Wishbone Suspension/Vehicle Adapter ==
  Veh : Inport
  Bus Creator3 : BusCreator  Inputs=2
  Bus Selector1 : BusSelector  OutputSignals=InertFrm.FrntAxl.Lft.Disp.X,InertFrm.FrntAxl.Lft.Disp.Y,InertFrm.FrntAxl.Lft.Disp.Z,InertFrm.FrntAxl.Rght.Disp.X,InertFrm.FrntAxl.Rght.Disp.Y,InertFrm.FrntAxl.Rght.Disp.Z,InertFrm.RearAxl.Lft.Disp.X,InertFrm.RearAxl.Lft.Disp.Y,InertFrm.RearAxl.Lft.Disp.Z,InertFrm.RearAxl.Rght.Disp.X,InertFrm.RearAxl.Rght.Disp.Y,InertFrm.RearAxl.Rght.Disp.Z
  Bus Selector2 : BusSelector  OutputSignals=BdyFrm.FrntAxl.Lft.Vel.xdot,BdyFrm.FrntAxl.Lft.Vel.ydot,BdyFrm.FrntAxl.Lft.Vel.zdot,BdyFrm.FrntAxl.Rght.Vel.xdot,BdyFrm.FrntAxl.Rght.Vel.ydot,BdyFrm.FrntAxl.Rght.Vel.zdot,BdyFrm.RearAxl.Lft.Vel.xdot,BdyFrm.RearAxl.Lft.Vel.ydot,BdyFrm.RearAxl.Lft.Vel.zdot,BdyFrm.RearAxl.Rght.Vel.xdot,BdyFrm.RearAxl.Rght.Vel.ydot,BdyFrm.RearAxl.Rght.Vel.zdot
  Inertial Frame CG to Axle Offset : Constant  Value=[zeros(2,4);h*ones(1,4)+VEH.InitialVertPosition*0]
  Mux1 : Mux  Inputs=12
  Mux2 : Mux  Inputs=12
  Reshape1 : Reshape  OutputDimensionality=Customize  OutputDimensions=[3,4]
  Reshape2 : Reshape  OutputDimensionality=Customize  OutputDimensions=[3,4]
  Sum : Sum  Inputs=|+-
  VehSusp : Outport  VectorParamsAs1DForOutWhenUnconnected=off
  wires:
  Reshape2/1 -> Bus Creator3/2  "V"
  Bus Creator3/1 -> VehSusp/1  "Veh"
  Bus Selector1/1 -> Mux2/1  "<X>"
  Bus Selector1/2 -> Mux2/2  "<Y>"
  Bus Selector1/3 -> Mux2/3  "<Z>"
  Bus Selector1/4 -> Mux2/4  "<X>"
  Bus Selector1/5 -> Mux2/5  "<Y>"
  Bus Selector1/6 -> Mux2/6  "<Z>"
  Bus Selector1/7 -> Mux2/7  "<X>"
  Bus Selector1/8 -> Mux2/8  "<Y>"
  Bus Selector1/9 -> Mux2/9  "<Z>"
  Bus Selector1/10 -> Mux2/10  "<X>"
  Bus Selector1/11 -> Mux2/11  "<Y>"
  Bus Selector1/12 -> Mux2/12  "<Z>"
  Bus Selector2/1 -> Mux1/1  "<xdot>"
  Bus Selector2/2 -> Mux1/2  "<ydot>"
  Bus Selector2/3 -> Mux1/3  "<zdot>"
  Bus Selector2/4 -> Mux1/4  "<xdot>"
  Bus Selector2/5 -> Mux1/5  "<ydot>"
  Bus Selector2/6 -> Mux1/6  "<zdot>"
  Bus Selector2/7 -> Mux1/7  "<xdot>"
  Bus Selector2/8 -> Mux1/8  "<ydot>"
  Bus Selector2/9 -> Mux1/9  "<zdot>"
  Bus Selector2/10 -> Mux1/10  "<xdot>"
  Bus Selector2/11 -> Mux1/11  "<ydot>"
  Bus Selector2/12 -> Mux1/12  "<zdot>"
  Mux1/1 -> Reshape2/1
  Inertial Frame CG to Axle Offset/1 -> Sum/2
  Sum/1 -> Bus Creator3/1  "P"
  Veh/1 -> Bus Selector2/1, Bus Selector1/1
  Mux2/1 -> Reshape1/1
  Reshape1/1 -> Sum/1

== system car_system_SIL_PIL/Passenger Vehicle/Subsystem6/Suspension/Double Wishbone Suspension/Wheel  Adapter ==
  Wheels : Inport
  Bus Selector : BusSelector  OutputSignals=TireFrame.Fx,TireFrame.Fy
  Bus Selector1 : BusSelector  OutputSignals=TireFrame.Re
  Bus Selector2 : BusSelector  OutputSignals=TireFrame.Mx,TireFrame.My,TireFrame.Mz
  Bus Selector3 : BusSelector  OutputSignals=TireFrame.z,TireFrame.zdot
  Matrix Concatenate : Concatenate  NumInputs=3  Mode=Multidimensional array
  Reshape{,1..7} (8 alike) : Reshape  OutputDimensionality=Row vector (2-D)
  WhlFx : Outport  VectorParamsAs1DForOutWhenUnconnected=off
  WhlFy : Outport  Port=2  VectorParamsAs1DForOutWhenUnconnected=off
  z : Outport  Port=3  VectorParamsAs1DForOutWhenUnconnected=off
  zdot : Outport  Port=4  VectorParamsAs1DForOutWhenUnconnected=off
  M : Outport  Port=5  VectorParamsAs1DForOutWhenUnconnected=off
  Re : Outport  Port=6  VectorParamsAs1DForOutWhenUnconnected=off
  wires:
  Reshape7/1 -> WhlFy/1
  Reshape6/1 -> WhlFx/1
  Bus Selector/1 -> Reshape6/1  "<Fx>"
  Bus Selector/2 -> Reshape7/1  "<Fy>"
  Bus Selector3/1 -> Reshape/1  "<z>"
  Wheels/1 -> Bus Selector1/1, Bus Selector2/1, Bus Selector3/1, Bus Selector/1
  Bus Selector3/2 -> Reshape2/1  "<zdot>"
  Reshape2/1 -> zdot/1  "zdot"
  Bus Selector1/1 -> Reshape1/1  "<Re>"
  Reshape1/1 -> Re/1  "Re"
  Bus Selector2/1 -> Reshape3/1  "<Mx>"
  Bus Selector2/2 -> Reshape4/1  "<My>"
  Bus Selector2/3 -> Reshape5/1  "<Mz>"
  Reshape3/1 -> Matrix Concatenate/1
  Reshape4/1 -> Matrix Concatenate/2
  Reshape5/1 -> Matrix Concatenate/3
  Matrix Concatenate/1 -> M/1  "M"
  Reshape/1 -> z/1  "z"

== system car_system_SIL_PIL/Passenger Vehicle/Subsystem6/Suspension/Independent Mapped Front Suspension Mapped Solid Axle Rear Suspension/Steer Rate Adapter ==
  Veh : Inport
  Add : Sum
  Bus Selector3 : BusSelector  OutputSignals=BdyFrm.Cg.AngVel.r
  Constant : Constant  Value=zeros(1,4)
  Matrix Concatenate : Concatenate  NumInputs=3  Mode=Multidimensional array
  Matrix Concatenate1 : Concatenate  NumInputs=3  Mode=Multidimensional array
  Reshape2 : Reshape  OutputDimensionality=Row vector (2-D)
  Reshape3 : Reshape  OutputDimensionality=Row vector (2-D)
  Reshape4 : Reshape  OutputDimensionality=Row vector (2-D)
  Selector3 : Selector  InputPortWidth=1  IndexOptions=Index vector (dialog)  Indices=[1 1 1 1]  OutputSizes=1
  SteerRates : Constant  Value=zeros(1,4)
  AngVel : Outport  VectorParamsAs1DForOutWhenUnconnected=off
  wires:
  Reshape2/1 -> Matrix Concatenate1/1, Matrix Concatenate1/3, Matrix Concatenate1/2
  Constant/1 -> Reshape3/1
  Selector3/1 -> Reshape4/1
  Bus Selector3/1 -> Selector3/1  "<r>"
  Matrix Concatenate/1 -> Add/2
  SteerRates/1 -> Reshape2/1
  Reshape4/1 -> Matrix Concatenate/3
  Reshape3/1 -> Matrix Concatenate/2, Matrix Concatenate/1
  Matrix Concatenate1/1 -> Add/1
  Veh/1 -> Bus Selector3/1
  Add/1 -> AngVel/1  "AngVel"

== system car_system_SIL_PIL/Passenger Vehicle/Subsystem6/Suspension/Independent Mapped Front Suspension Mapped Solid Axle Rear Suspension/Steering Adapter ==
  Steer : Inport
  Reshape1 : Reshape  OutputDimensionality=Row vector (2-D)
  Selector : Selector  IndexOptions=Index vector (dialog)  Indices=[1 2]  OutputSizes=1
  StrgAng : Outport  VectorParamsAs1DForOutWhenUnconnected=off
  wires:
  Reshape1/1 -> StrgAng/1
  Steer/1 -> Selector/1
  Selector/1 -> Reshape1/1

== system car_system_SIL_PIL/Passenger Vehicle/Subsystem6/Suspension/Independent Mapped Front Suspension Mapped Solid Axle Rear Suspension/Vehicle Adapter ==
  Veh : Inport
  Bus Creator3 : BusCreator  Inputs=2
  Bus Selector1 : BusSelector  OutputSignals=InertFrm.FrntAxl.Lft.Disp.X,InertFrm.FrntAxl.Lft.Disp.Y,InertFrm.FrntAxl.Lft.Disp.Z,InertFrm.FrntAxl.Rght.Disp.X,InertFrm.FrntAxl.Rght.Disp.Y,InertFrm.FrntAxl.Rght.Disp.Z,InertFrm.RearAxl.Lft.Disp.X,InertFrm.RearAxl.Lft.Disp.Y,InertFrm.RearAxl.Lft.Disp.Z,InertFrm.RearAxl.Rght.Disp.X,InertFrm.RearAxl.Rght.Disp.Y,InertFrm.RearAxl.Rght.Disp.Z
  Bus Selector2 : BusSelector  OutputSignals=BdyFrm.FrntAxl.Lft.Vel.xdot,BdyFrm.FrntAxl.Lft.Vel.ydot,BdyFrm.FrntAxl.Lft.Vel.zdot,BdyFrm.FrntAxl.Rght.Vel.xdot,BdyFrm.FrntAxl.Rght.Vel.ydot,BdyFrm.FrntAxl.Rght.Vel.zdot,BdyFrm.RearAxl.Lft.Vel.xdot,BdyFrm.RearAxl.Lft.Vel.ydot,BdyFrm.RearAxl.Lft.Vel.zdot,BdyFrm.RearAxl.Rght.Vel.xdot,BdyFrm.RearAxl.Rght.Vel.ydot,BdyFrm.RearAxl.Rght.Vel.zdot
  Inertial Frame CG to Axle Offset : Constant  Value=[zeros(2,4);h*ones(1,4)]
  Mux1 : Mux  Inputs=12
  Mux2 : Mux  Inputs=12
  Reshape : Reshape  OutputDimensionality=Customize  OutputDimensions=[3,4]
  Reshape2 : Reshape  OutputDimensionality=Customize  OutputDimensions=[3,4]
  Sum : Sum  Inputs=|+-
  VehSusp : Outport  VectorParamsAs1DForOutWhenUnconnected=off
  wires:
  Veh/1 -> Bus Selector2/1, Bus Selector1/1
  Reshape2/1 -> Bus Creator3/2  "V"
  Bus Creator3/1 -> VehSusp/1  "Veh"
  Reshape/1 -> Sum/1
  Bus Selector1/1 -> Mux2/1  "<X>"
  Bus Selector1/2 -> Mux2/2  "<Y>"
  Bus Selector1/3 -> Mux2/3  "<Z>"
  Bus Selector1/4 -> Mux2/4  "<X>"
  Bus Selector1/5 -> Mux2/5  "<Y>"
  Bus Selector1/6 -> Mux2/6  "<Z>"
  Bus Selector1/7 -> Mux2/7  "<X>"
  Bus Selector1/8 -> Mux2/8  "<Y>"
  Bus Selector1/9 -> Mux2/9  "<Z>"
  Bus Selector1/10 -> Mux2/10  "<X>"
  Bus Selector1/11 -> Mux2/11  "<Y>"
  Bus Selector1/12 -> Mux2/12  "<Z>"
  Bus Selector2/1 -> Mux1/1  "<xdot>"
  Bus Selector2/2 -> Mux1/2  "<ydot>"
  Bus Selector2/3 -> Mux1/3  "<zdot>"
  Bus Selector2/4 -> Mux1/4  "<xdot>"
  Bus Selector2/5 -> Mux1/5  "<ydot>"
  Bus Selector2/6 -> Mux1/6  "<zdot>"
  Bus Selector2/7 -> Mux1/7  "<xdot>"
  Bus Selector2/8 -> Mux1/8  "<ydot>"
  Bus Selector2/9 -> Mux1/9  "<zdot>"
  Bus Selector2/10 -> Mux1/10  "<xdot>"
  Bus Selector2/11 -> Mux1/11  "<ydot>"
  Bus Selector2/12 -> Mux1/12  "<zdot>"
  Mux1/1 -> Reshape2/1
  Mux2/1 -> Reshape/1
  Inertial Frame CG to Axle Offset/1 -> Sum/2
  Sum/1 -> Bus Creator3/1  "P"

== system car_system_SIL_PIL/Passenger Vehicle/Subsystem6/Suspension/Independent Mapped Front Suspension Mapped Solid Axle Rear Suspension/Wheel  Adapter ==
  Wheels : Inport
  Bus Selector : BusSelector  OutputSignals=TireFrame.Fx,TireFrame.Fy
  Bus Selector1 : BusSelector  OutputSignals=TireFrame.Re
  Bus Selector2 : BusSelector  OutputSignals=TireFrame.Mx,TireFrame.My,TireFrame.Mz
  Bus Selector3 : BusSelector  OutputSignals=TireFrame.z,TireFrame.zdot
  Matrix Concatenate : Concatenate  NumInputs=3  Mode=Multidimensional array
  Reshape{,1..7} (8 alike) : Reshape  OutputDimensionality=Row vector (2-D)
  WhlFx : Outport  VectorParamsAs1DForOutWhenUnconnected=off
  WhlFy : Outport  Port=2  VectorParamsAs1DForOutWhenUnconnected=off
  z : Outport  Port=3  VectorParamsAs1DForOutWhenUnconnected=off
  zdot : Outport  Port=4  VectorParamsAs1DForOutWhenUnconnected=off
  M : Outport  Port=5  VectorParamsAs1DForOutWhenUnconnected=off
  Re : Outport  Port=6  VectorParamsAs1DForOutWhenUnconnected=off
  wires:
  Reshape7/1 -> WhlFy/1
  Reshape6/1 -> WhlFx/1
  Bus Selector/1 -> Reshape6/1  "<Fx>"
  Bus Selector/2 -> Reshape7/1  "<Fy>"
  Bus Selector3/1 -> Reshape/1  "<z>"
  Wheels/1 -> Bus Selector1/1, Bus Selector2/1, Bus Selector3/1, Bus Selector/1
  Bus Selector3/2 -> Reshape2/1  "<zdot>"
  Reshape2/1 -> zdot/1  "zdot"
  Bus Selector1/1 -> Reshape1/1  "<Re>"
  Reshape1/1 -> Re/1  "Re"
  Bus Selector2/1 -> Reshape3/1  "<Mx>"
  Bus Selector2/2 -> Reshape4/1  "<My>"
  Bus Selector2/3 -> Reshape5/1  "<Mz>"
  Reshape3/1 -> Matrix Concatenate/1
  Reshape4/1 -> Matrix Concatenate/2
  Reshape5/1 -> Matrix Concatenate/3
  Matrix Concatenate/1 -> M/1  "M"
  Reshape/1 -> z/1  "z"

== system car_system_SIL_PIL/Passenger Vehicle/Subsystem6/Suspension/MacPherson Front Suspension Solid Axle Rear Suspension/Steer Rate Adapter ==
  Veh : Inport
  Add : Sum
  Bus Selector3 : BusSelector  OutputSignals=BdyFrm.Cg.AngVel.r
  Constant : Constant  Value=zeros(1,4)
  Matrix Concatenate : Concatenate  NumInputs=3  Mode=Multidimensional array
  Matrix Concatenate1 : Concatenate  NumInputs=3  Mode=Multidimensional array
  Reshape2 : Reshape  OutputDimensionality=Row vector (2-D)
  Reshape3 : Reshape  OutputDimensionality=Row vector (2-D)
  Reshape4 : Reshape  OutputDimensionality=Row vector (2-D)
  Selector3 : Selector  InputPortWidth=1  IndexOptions=Index vector (dialog)  Indices=[1 1 1 1]  OutputSizes=1
  SteerRates : Constant  Value=zeros(1,4)
  AngVel : Outport  VectorParamsAs1DForOutWhenUnconnected=off
  wires:
  Reshape2/1 -> Matrix Concatenate1/1, Matrix Concatenate1/3, Matrix Concatenate1/2
  Constant/1 -> Reshape3/1
  Selector3/1 -> Reshape4/1
  Bus Selector3/1 -> Selector3/1  "<r>"
  Matrix Concatenate/1 -> Add/2
  SteerRates/1 -> Reshape2/1
  Reshape4/1 -> Matrix Concatenate/3
  Reshape3/1 -> Matrix Concatenate/2, Matrix Concatenate/1
  Matrix Concatenate1/1 -> Add/1
  Veh/1 -> Bus Selector3/1
  Add/1 -> AngVel/1  "AngVel"

== system car_system_SIL_PIL/Passenger Vehicle/Subsystem6/Suspension/MacPherson Front Suspension Solid Axle Rear Suspension/Steering Adapter ==
  Steer : Inport
  Reshape1 : Reshape  OutputDimensionality=Row vector (2-D)
  Selector : Selector  IndexOptions=Index vector (dialog)  Indices=[1 2]  OutputSizes=1
  StrgAng : Outport  VectorParamsAs1DForOutWhenUnconnected=off
  wires:
  Reshape1/1 -> StrgAng/1
  Steer/1 -> Selector/1
  Selector/1 -> Reshape1/1

== system car_system_SIL_PIL/Passenger Vehicle/Subsystem6/Suspension/MacPherson Front Suspension Solid Axle Rear Suspension/Vehicle Adapter ==
  Veh : Inport
  Bus Creator3 : BusCreator  Inputs=2
  Bus Selector1 : BusSelector  OutputSignals=InertFrm.FrntAxl.Lft.Disp.X,InertFrm.FrntAxl.Lft.Disp.Y,InertFrm.FrntAxl.Lft.Disp.Z,InertFrm.FrntAxl.Rght.Disp.X,InertFrm.FrntAxl.Rght.Disp.Y,InertFrm.FrntAxl.Rght.Disp.Z,InertFrm.RearAxl.Lft.Disp.X,InertFrm.RearAxl.Lft.Disp.Y,InertFrm.RearAxl.Lft.Disp.Z,InertFrm.RearAxl.Rght.Disp.X,InertFrm.RearAxl.Rght.Disp.Y,InertFrm.RearAxl.Rght.Disp.Z
  Bus Selector2 : BusSelector  OutputSignals=BdyFrm.FrntAxl.Lft.Vel.xdot,BdyFrm.FrntAxl.Lft.Vel.ydot,BdyFrm.FrntAxl.Lft.Vel.zdot,BdyFrm.FrntAxl.Rght.Vel.xdot,BdyFrm.FrntAxl.Rght.Vel.ydot,BdyFrm.FrntAxl.Rght.Vel.zdot,BdyFrm.RearAxl.Lft.Vel.xdot,BdyFrm.RearAxl.Lft.Vel.ydot,BdyFrm.RearAxl.Lft.Vel.zdot,BdyFrm.RearAxl.Rght.Vel.xdot,BdyFrm.RearAxl.Rght.Vel.ydot,BdyFrm.RearAxl.Rght.Vel.zdot
  Inertial Frame CG to Axle Offset : Constant  Value=[zeros(2,4);h*ones(1,4)]
  Mux1 : Mux  Inputs=12
  Mux2 : Mux  Inputs=12
  Reshape : Reshape  OutputDimensionality=Customize  OutputDimensions=[3,4]
  Reshape2 : Reshape  OutputDimensionality=Customize  OutputDimensions=[3,4]
  Sum : Sum  Inputs=|+-
  VehSusp : Outport  VectorParamsAs1DForOutWhenUnconnected=off
  wires:
  Veh/1 -> Bus Selector2/1, Bus Selector1/1
  Reshape2/1 -> Bus Creator3/2  "V"
  Bus Creator3/1 -> VehSusp/1  "Veh"
  Reshape/1 -> Sum/1
  Bus Selector1/1 -> Mux2/1  "<X>"
  Bus Selector1/2 -> Mux2/2  "<Y>"
  Bus Selector1/3 -> Mux2/3  "<Z>"
  Bus Selector1/4 -> Mux2/4  "<X>"
  Bus Selector1/5 -> Mux2/5  "<Y>"
  Bus Selector1/6 -> Mux2/6  "<Z>"
  Bus Selector1/7 -> Mux2/7  "<X>"
  Bus Selector1/8 -> Mux2/8  "<Y>"
  Bus Selector1/9 -> Mux2/9  "<Z>"
  Bus Selector1/10 -> Mux2/10  "<X>"
  Bus Selector1/11 -> Mux2/11  "<Y>"
  Bus Selector1/12 -> Mux2/12  "<Z>"
  Bus Selector2/1 -> Mux1/1  "<xdot>"
  Bus Selector2/2 -> Mux1/2  "<ydot>"
  Bus Selector2/3 -> Mux1/3  "<zdot>"
  Bus Selector2/4 -> Mux1/4  "<xdot>"
  Bus Selector2/5 -> Mux1/5  "<ydot>"
  Bus Selector2/6 -> Mux1/6  "<zdot>"
  Bus Selector2/7 -> Mux1/7  "<xdot>"
  Bus Selector2/8 -> Mux1/8  "<ydot>"
  Bus Selector2/9 -> Mux1/9  "<zdot>"
  Bus Selector2/10 -> Mux1/10  "<xdot>"
  Bus Selector2/11 -> Mux1/11  "<ydot>"
  Bus Selector2/12 -> Mux1/12  "<zdot>"
  Mux1/1 -> Reshape2/1
  Mux2/1 -> Reshape/1
  Inertial Frame CG to Axle Offset/1 -> Sum/2
  Sum/1 -> Bus Creator3/1  "P"

== system car_system_SIL_PIL/Passenger Vehicle/Subsystem6/Suspension/MacPherson Front Suspension Solid Axle Rear Suspension/Wheel  Adapter ==
  Wheels : Inport
  Bus Selector : BusSelector  OutputSignals=TireFrame.Fx,TireFrame.Fy
  Bus Selector1 : BusSelector  OutputSignals=TireFrame.Re
  Bus Selector2 : BusSelector  OutputSignals=TireFrame.Mx,TireFrame.My,TireFrame.Mz
  Bus Selector3 : BusSelector  OutputSignals=TireFrame.z,TireFrame.zdot
  Matrix Concatenate : Concatenate  NumInputs=3  Mode=Multidimensional array
  Reshape{,1..7} (8 alike) : Reshape  OutputDimensionality=Row vector (2-D)
  WhlFx : Outport  VectorParamsAs1DForOutWhenUnconnected=off
  WhlFy : Outport  Port=2  VectorParamsAs1DForOutWhenUnconnected=off
  z : Outport  Port=3  VectorParamsAs1DForOutWhenUnconnected=off
  zdot : Outport  Port=4  VectorParamsAs1DForOutWhenUnconnected=off
  M : Outport  Port=5  VectorParamsAs1DForOutWhenUnconnected=off
  Re : Outport  Port=6  VectorParamsAs1DForOutWhenUnconnected=off
  wires:
  Reshape7/1 -> WhlFy/1
  Reshape6/1 -> WhlFx/1
  Bus Selector/1 -> Reshape6/1  "<Fx>"
  Bus Selector/2 -> Reshape7/1  "<Fy>"
  Bus Selector3/1 -> Reshape/1  "<z>"
  Wheels/1 -> Bus Selector1/1, Bus Selector2/1, Bus Selector3/1, Bus Selector/1
  Bus Selector3/2 -> Reshape2/1  "<zdot>"
  Reshape2/1 -> zdot/1  "zdot"
  Bus Selector1/1 -> Reshape1/1  "<Re>"
  Reshape1/1 -> Re/1  "Re"
  Bus Selector2/1 -> Reshape3/1  "<Mx>"
  Bus Selector2/2 -> Reshape4/1  "<My>"
  Bus Selector2/3 -> Reshape5/1  "<Mz>"
  Reshape3/1 -> Matrix Concatenate/1
  Reshape4/1 -> Matrix Concatenate/2
  Reshape5/1 -> Matrix Concatenate/3
  Matrix Concatenate/1 -> M/1  "M"
  Reshape/1 -> z/1  "z"

== system car_system_SIL_PIL/Passenger Vehicle/Subsystem6/Suspension/MacPherson Suspension/Steer Rate Adapter ==
  Veh : Inport
  Add : Sum
  Bus Selector3 : BusSelector  OutputSignals=BdyFrm.Cg.AngVel.r
  Constant : Constant  Value=zeros(1,4)
  Matrix Concatenate : Concatenate  NumInputs=3  Mode=Multidimensional array
  Matrix Concatenate1 : Concatenate  NumInputs=3  Mode=Multidimensional array
  Reshape2 : Reshape  OutputDimensionality=Row vector (2-D)
  Reshape3 : Reshape  OutputDimensionality=Row vector (2-D)
  Reshape4 : Reshape  OutputDimensionality=Row vector (2-D)
  Selector3 : Selector  InputPortWidth=1  IndexOptions=Index vector (dialog)  Indices=[1 1 1 1]  OutputSizes=1
  SteerRates : Constant  Value=zeros(1,4)
  AngVel : Outport  VectorParamsAs1DForOutWhenUnconnected=off
  wires:
  Reshape2/1 -> Matrix Concatenate1/1, Matrix Concatenate1/3, Matrix Concatenate1/2
  Constant/1 -> Reshape3/1
  Selector3/1 -> Reshape4/1
  Bus Selector3/1 -> Selector3/1  "<r>"
  Matrix Concatenate/1 -> Add/2
  SteerRates/1 -> Reshape2/1
  Reshape4/1 -> Matrix Concatenate/3
  Reshape3/1 -> Matrix Concatenate/2, Matrix Concatenate/1
  Matrix Concatenate1/1 -> Add/1
  Veh/1 -> Bus Selector3/1
  Add/1 -> AngVel/1  "AngVel"
